simulink model "controller"  (R2021b)
settings: Solver=ode4  StartTime=0.0  StopTime=10.0  FixedStep=0.001  RelTol=1e-3
undefined symbols (not defined in the file): B, J, K2, K3, Kb, Kt, L, L1, L2, L3, R, Ts
settings Model: Creator=user  LastModifiedBy=user

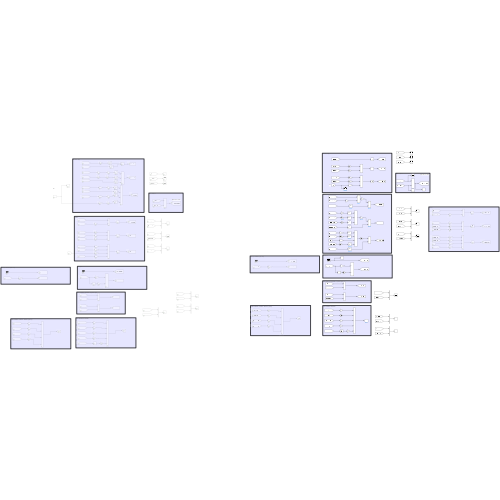
[thumbnail: Simulink's stored preview of the top-level diagram]
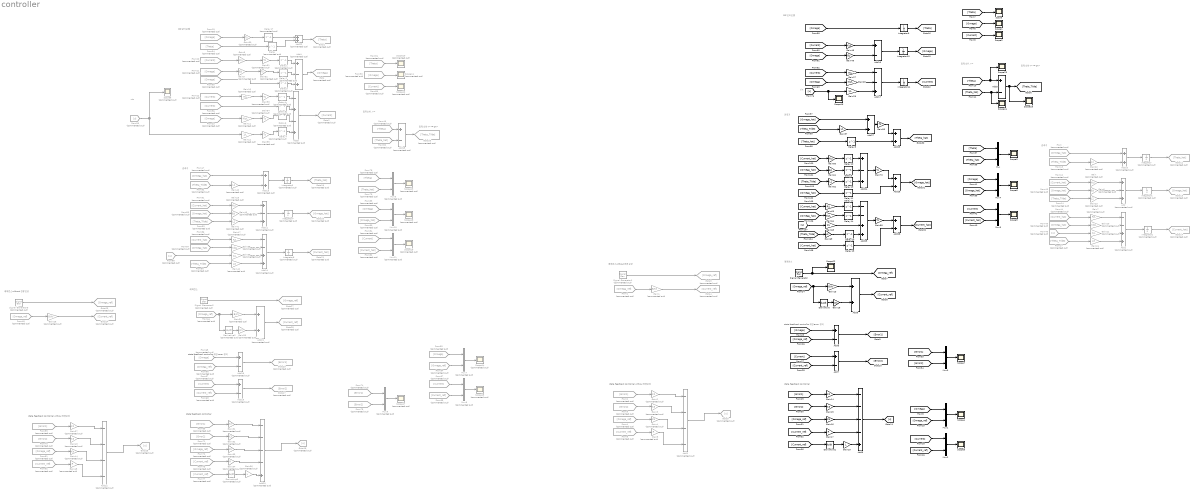
== system controller ==
  note: 관측기
  note: vin
  note: DC 모터 모델
  note: state feedback controller
  note: 레퍼런스
  note: state feedback controller 위한 error 정의
  note: 레퍼런스 without 전류 보상
  note: state feedback controller without 전류보상
  note: 출력 오차 Y~ = CX~
  note: 출력 오차, Y~
  note: 관측기
  note: vin
  note: state feedback controller
  note: 관측기
  note: 출력 오차 Y~ = CX~
  note: 레퍼런스 without 전류 보상
  note: 출력 오차, Y~
  note: DC 모터 모델
  note: state feedback controller without 전류보상
  note: state feedback controller 위한 error 정의
  note: 레퍼런스
  Add : Sum  Commented=on  Inputs=+-+
  Add1 : Sum  Commented=on  Inputs=----
  Add{10,13,21..22} (4 alike) : Sum  Commented=on
  Add11 : Sum  Commented=on  Inputs=+-+
  Add12 : Sum  Commented=on  Inputs=----
  Add14 : Sum  Commented=on  Inputs=--++
  Add15 : Sum  Commented=on  Inputs=+-
  Add{3,6..7,16} (4 alike) : Sum  Inputs=+-
  Add17 : Sum  Inputs=--+
  Add18 : Sum  Commented=on  Inputs=+-
  Add19 : Sum  Commented=on  Inputs=+-
  Add2 : Sum  Commented=on  Inputs=--++
  Add20 : Sum  Commented=on  Inputs=----+
  Add{9,23,26..28} (5 alike) : Sum
  Add24 : Sum  Inputs=+-+
  Add25 : Sum  Inputs=--++
  Add4 : Sum  Commented=on  Inputs=+-+
  Add5 : Sum  Commented=on  Inputs=-+-+
  Add8 : Sum  Inputs=----+
  Delay : Delay  Commented=on  DelayLength=1  InitialCondition=0
  Delay{1..7,17} (8 alike) : Delay  Commented=on  DelayLength=1
  Delay{8..14,19..20} (9 alike) : Delay  DelayLength=1
  Derivative : Derivative
  Derivative1 : Derivative
  Derivative2 : Derivative  Commented=on
  Derivative3 : Derivative  Commented=on
  From{,43,45,47,80,85,87} (7 alike) : From  Commented=on  GotoTag=Omega_hat
  From{1,4,48,54,64,66,72,81} (8 alike) : From  Commented=on  GotoTag=Omega_ref
  From{12,44,51,82,86} (5 alike) : From  Commented=on  GotoTag=Current_hat
  From{13..14,17,52..53,56} (6 alike) : From  Commented=on  GotoTag=Theta_Tilde
  From{19,21,23,65,83,90,93,95} (8 alike) : From  Commented=on  GotoTag=Omega
  From{2,59,69,74} (4 alike) : From  Commented=on  GotoTag=Error1
  From{20,22,57,67,84,89,96} (7 alike) : From  Commented=on  GotoTag=Current
  From{3,70..71,75} (4 alike) : From  Commented=on  GotoTag=Error2
  From35 : From  Commented=on  GotoTag=u
  From46 : From  Commented=on  GotoTag=u
  From{49,78,91,94} (4 alike) : From  Commented=on  GotoTag=Theta
  From50 : From  Commented=on  GotoTag=Theta_hat
  From{8,55,68,73,77,92} (6 alike) : From  Commented=on  GotoTag=Current_ref
  From79 : From  Commented=on  GotoTag=Theta_hat
  From88 : From  Commented=on  GotoTag=u
  Gain : Gain  Commented=on  Gain=Kt/J
  Gain1 : Gain  Commented=on  Gain=B/Kt
  Gain10 : Gain  Commented=on  Gain=R/L
  Gain11 : Gain  Commented=on  Gain=Kb/L
  Gain12 : Gain  Commented=on  Gain=1/L
  Gain13 : Gain  Gain=B/Kt
  Gain14 : Gain  Gain=K2
  Gain15 : Gain  Gain=K3
  Gain16 : Gain  Gain=Kb
  Gain17 : Gain  Gain=R
  Gain18 : Gain  Gain=J/Kt
  Gain19 : Gain  Gain=L
  Gain2 : Gain  Commented=on  Gain=K2
  Gain20 : Gain  Commented=on  Gain=Kb/L
  Gain21 : Gain  Commented=on  Gain=1/L
  Gain22 : Gain  Commented=on  Gain=L1
  Gain23 : Gain  Commented=on  Gain=L2
  Gain24 : Gain  Commented=on  Gain=L3
  Gain25 : Gain  Commented=on  Gain=Kt/J
  Gain26 : Gain  Commented=on  Gain=B/Kt
  Gain27 : Gain  Gain=R/L
  Gain28 : Gain  Gain=Kb/L
  Gain29 : Gain  Gain=1/L
  Gain3 : Gain  Commented=on  Gain=K3
  Gain30 : Gain  Commented=on  Gain=B/Kt
  Gain31 : Gain  Commented=on  Gain=K2
  Gain32 : Gain  Commented=on  Gain=K3
  Gain33 : Gain  Commented=on  Gain=Kb
  Gain34 : Gain  Commented=on  Gain=R
  Gain35 : Gain  Commented=on  Gain=J/Kt
  Gain36 : Gain  Commented=on  Gain=L
  Gain37 : Gain  Commented=on  Gain=K2
  Gain38 : Gain  Commented=on  Gain=Kb/L
  Gain39 : Gain  Commented=on  Gain=1/L
  Gain4 : Gain  Commented=on  Gain=Kb
  Gain40 : Gain  Commented=on  Gain=L1
  Gain41 : Gain  Commented=on  Gain=L2
  Gain42 : Gain  Commented=on  Gain=L3
  Gain43 : Gain  Commented=on  Gain=K3
  Gain44 : Gain  Commented=on  Gain=Kb
  Gain45 : Gain  Commented=on  Gain=R
  Gain46 : Gain  Commented=on  Gain=B/J
  Gain47 : Gain  Commented=on  Gain=R/L
  Gain48 : Gain  Gain=Kt/J
  Gain49 : Gain  Gain=B/J
  Gain5 : Gain  Commented=on  Gain=R
  Gain{50..55} (6 alike) : Gain  Commented=on  Gain=Ts
  Gain56 : Gain  Gain=Ts
  Gain57 : Gain  Gain=L1
  Gain58 : Gain  Gain=Ts
  Gain6 : Gain  Commented=on  Gain=B/J
  Gain60 : Gain  Gain=Kt/J
  Gain61 : Gain  Gain=B/J
  Gain62 : Gain  Gain=L2
  Gain63 : Gain  Gain=R/L
  Gain64 : Gain  Gain=Kb/L
  Gain65 : Gain  Gain=1/L
  Gain69 : Gain  Gain=L3
  Gain7 : Gain  Commented=on  Gain=R/L
  Gain70 : Gain  Gain=Ts
  Gain8 : Gain  Commented=on  Gain=Kt/J
  Gain9 : Gain  Commented=on  Gain=B/J
  Goto : Goto  Commented=on  GotoTag=Omega
  Goto1 : Goto  Commented=on  GotoTag=Theta
  Goto12 : Goto  Commented=on  GotoTag=Theta_hat
  Goto13 : Goto  Commented=on  GotoTag=Omega_hat
  Goto14 : Goto  Commented=on  GotoTag=Current_hat
  Goto17 : Goto  Commented=on  GotoTag=Error2
  Goto18 : Goto  Commented=on  GotoTag=u
  Goto19 : Goto  Commented=on  GotoTag=Theta_hat
  Goto2 : Goto  Commented=on  GotoTag=Current
  Goto20 : Goto  Commented=on  GotoTag=Omega_hat
  Goto21 : Goto  Commented=on  GotoTag=Current_hat
  Goto23 : Goto  Commented=on  GotoTag=Omega_ref
  Goto24 : Goto  Commented=on  GotoTag=Current_ref
  Goto25 : Goto  Commented=on  GotoTag=u
  Goto26 : Goto  Commented=on  GotoTag=Theta_Tilde
  Goto27 : Goto  Commented=on  GotoTag=Omega_ref
  Goto28 : Goto  Commented=on  GotoTag=Current_ref
  Goto29 : Goto  Commented=on  GotoTag=Error1
  Goto3 : Goto  Commented=on  GotoTag=Omega_ref
  Goto4 : Goto  Commented=on  GotoTag=Current_ref
  Goto5 : Goto  Commented=on  GotoTag=u
  Integrator{,1..2,6..8} (6 alike) : Integrator  Commented=on
  Integrator10 : Integrator
  Integrator11 : Integrator
  Integrator9 : Integrator  InitialCondition=1
  Mux{,1..5} (6 alike) : Mux  Inputs=2
  Mux{6..11} (6 alike) : Mux  Commented=on  Inputs=2
  Scope{,1..5,7..9,16,22..25} (14 alike) : Scope
  Scope{6,10..15,17..19} (10 alike) : Scope  Commented=on
  Signal Generator : SignalGenerator  Units=rad/sec
  Signal Generator1 : SignalGenerator  Commented=on  Units=rad/sec
  Signal Generator2 : SignalGenerator  Commented=on  Units=rad/sec
  Signal Generator3 : SignalGenerator  Commented=on  Units=rad/sec
  wires:
  Add22/1 -> Goto1/1
  From19/1 -> Gain50/1
  From23/1 -> Gain11/1
  From20/1 -> Gain8/1
  From21/1 -> Gain9/1
  From22/1 -> Gain10/1
  Gain8/1 -> Gain51/1
  Gain9/1 -> Gain52/1
  [Current] -> Scope2/1
  [Omega] -> Scope1/1
  [Theta] -> Scope/1
  From35/1 -> Scope6/1, Gain12/1
  [Current_ref] -> Derivative1/1
  Gain19/1 -> Add8/5
  Derivative1/1 -> Gain19/1
  Gain17/1 -> Add8/4
  [Omega_ref] -> Add6/2
  [Current] -> Add7/1
  Gain18/1 -> Add9/2
  Mux3/1 -> Scope7/1
  Gain13/1 -> Add9/1
  [Omega_ref] -> Gain13/1, Derivative/1
  [Error1] -> Gain14/1
  Add9/1 -> [Current_ref]
  Derivative/1 -> Gain18/1
  Signal Generator/1 -> Scope22/1, [Omega_ref]
  [Error1] -> Mux3/1
  Gain16/1 -> Add8/3
  [Error2] -> Mux3/2
  [Error2] -> Gain15/1
  Add8/1 -> [u]
  Gain14/1 -> Add8/1
  [Current_ref] -> Gain17/1
  Add6/1 -> [Error1]
  Gain15/1 -> Add8/2
  [Omega_ref] -> Gain16/1
  [Current_ref] -> Add7/2
  Add7/1 -> [Error2]
  [Omega] -> Add6/1
  [Current] -> Mux2/1
  Mux2/1 -> Scope5/1
  [Current_ref] -> Mux2/2
  [Omega_ref] -> Mux1/2
  Mux1/1 -> Scope4/1
  Signal Generator1/1 -> Goto3/1
  From1/1 -> Gain1/1
  Gain1/1 -> Goto4/1
  Gain3/1 -> Add1/2
  From8/1 -> Gain5/1
  From4/1 -> Gain4/1
  From3/1 -> Gain3/1
  Add1/1 -> Goto5/1
  Gain2/1 -> Add1/1
  Gain4/1 -> Add1/3
  From2/1 -> Gain2/1
  Gain5/1 -> Add1/4
  [Omega] -> Mux1/1
  [Theta] -> Scope23/1, Add3/1
  [Theta_hat] -> Scope24/1, Add3/2
  [Theta_hat] -> Mux/2
  [Theta] -> Mux/1
  Gain6/1 -> Add/2
  Mux4/1 -> Scope8/1
  [Current_hat] -> Mux5/2
  Gain24/1 -> Add2/4
  Gain22/1 -> Add10/2
  Mux5/1 -> Scope9/1
  Gain23/1 -> Add/3
  [Omega] -> Mux4/1
  From/1 -> Add10/1
  From14/1 -> Gain23/1
  Integrator2/1 -> Goto14/1
  Add10/1 -> Integrator/1
  Integrator1/1 -> Goto13/1
  Gain7/1 -> Add2/1
  From12/1 -> Gain/1
  Gain21/1 -> Add2/3
  Add/1 -> Integrator1/1
  Mux/1 -> Scope3/1
  Add2/1 -> Integrator2/1
  From44/1 -> Gain7/1
  From17/1 -> Gain24/1
  From13/1 -> Gain22/1
  From45/1 -> Gain20/1
  [Omega_hat] -> Mux4/2
  Gain/1 -> Add/1
  From43/1 -> Gain6/1
  [Current] -> Mux5/1
  Gain20/1 -> Add2/2
  Integrator/1 -> Goto12/1
  From46/1 -> Gain21/1
  Gain47/1 -> Add14/1
  From56/1 -> Gain42/1
  Gain49/1 -> Add16/2
  Add13/1 -> Integrator6/1
  From50/1 -> Add15/2
  Integrator7/1 -> Goto20/1
  Add16/1 -> Integrator10/1
  Gain36/1 -> Add20/5
  From55/1 -> Mux8/2
  Gain41/1 -> Add11/3
  Mux11/1 -> Scope19/1
  From81/1 -> Gain44/1
  Gain26/1 -> Goto24/1
  From82/1 -> Mux11/2
  Add20/1 -> Goto18/1
  From77/1 -> Derivative3/1
  Gain40/1 -> Add13/2
  From93/1 -> Mux7/1
  Gain42/1 -> Add14/4
  Gain46/1 -> Add11/2
  From70/1 -> Gain43/1
  Gain37/1 -> Add12/1
  Gain31/1 -> Add20/1
  From71/1 -> Gain32/1
  Add12/1 -> Goto25/1
  From48/1 -> Gain26/1
  From65/1 -> Add18/1
  From57/1 -> Mux8/1
  Gain27/1 -> Add17/1
  From75/1 -> Mux9/2
  From92/1 -> Gain45/1
  Gain43/1 -> Add12/2
  From54/1 -> Mux7/2
  Gain32/1 -> Add20/2
  Mux8/1 -> Scope15/1
  Add19/1 -> Goto17/1
  Add17/1 -> Integrator11/1
  Gain30/1 -> Add21/1
  Derivative3/1 -> Gain36/1
  Gain48/1 -> Add16/1
  Add18/1 -> Goto29/1
  Add21/1 -> Goto28/1
  Integrator11/1 -> [Current]
  [Omega] -> Gain28/1
  Gain28/1 -> Add17/2
  [Current] -> Gain48/1
  Gain29/1 -> Add17/3
  From91/1 -> Scope10/1
  Gain44/1 -> Add12/3
  From68/1 -> Add19/2
  Signal Generator2/1 -> Goto27/1
  Integrator9/1 -> [Theta]
  From72/1 -> Gain33/1
  Derivative2/1 -> Gain35/1
  From49/1 -> Add15/1
  Integrator6/1 -> Goto19/1
  Integrator10/1 -> [Omega]
  Signal Generator3/1 -> Goto23/1
  From89/1 -> Scope12/1
  Mux6/1 -> Scope13/1
  From78/1 -> Mux6/1
  From53/1 -> Gain41/1
  Gain35/1 -> Add21/2
  Gain45/1 -> Add12/4
  From59/1 -> Gain37/1
  From67/1 -> Add19/1
  From66/1 -> Add18/2
  Add11/1 -> Integrator7/1
  [u] -> Scope16/1, Gain29/1
  From84/1 -> Mux11/1
  [Omega] -> Integrator9/1
  From88/1 -> Gain39/1
  Mux10/1 -> Scope18/1
  [Omega] -> Gain49/1
  From52/1 -> Gain40/1
  From64/1 -> Gain30/1, Derivative2/1
  Integrator8/1 -> Goto21/1
  Gain39/1 -> Add14/3
  From51/1 -> Gain25/1
  From69/1 -> Gain31/1
  From87/1 -> Gain38/1
  From73/1 -> Gain34/1
  From90/1 -> Scope11/1
  [Current] -> Gain27/1
  Gain25/1 -> Add11/1
  Gain38/1 -> Add14/2
  From85/1 -> Gain46/1
  Mux7/1 -> Scope14/1
  From47/1 -> Add13/1
  From80/1 -> Mux10/2
  Gain33/1 -> Add20/3
  From79/1 -> Mux6/2
  From83/1 -> Mux10/1
  Gain34/1 -> Add20/4
  Add15/1 -> Goto26/1
  From86/1 -> Gain47/1
  Mux9/1 -> Scope17/1
  Add14/1 -> Integrator8/1
  From74/1 -> Mux9/1
  From94/1 -> Delay/1
  Delay/1 -> Add22/2
  From95/1 -> Delay3/1
  Gain52/1 -> Delay2/1
  Gain51/1 -> Delay1/1
  Delay1/1 -> Add4/1
  Delay2/1 -> Add4/2
  Delay3/1 -> Add4/3
  Add4/1 -> Goto/1
  Gain10/1 -> Gain53/1
  Gain53/1 -> Delay4/1
  From96/1 -> Delay5/1
  Gain11/1 -> Gain54/1
  Gain54/1 -> Delay6/1
  Gain12/1 -> Gain55/1
  Gain55/1 -> Delay7/1
  Delay4/1 -> Add5/1
  Delay5/1 -> Add5/2
  Delay6/1 -> Add5/3
  Delay7/1 -> Add5/4
  Add5/1 -> Goto2/1
  [Theta_hat] -> Delay8/1
  Delay8/1 -> Add23/2
  [Theta_Tilde] -> Gain57/1
  Add23/1 -> [Theta_hat]
  Add24/1 -> Gain70/1
  [Omega_hat] -> Gain61/1
  [Omega_hat] -> Delay11/1
  [Current_hat] -> Gain60/1
  [Theta_Tilde] -> Gain62/1
  [Current_hat] -> Gain63/1
  [Omega_hat] -> Gain64/1
  [Theta_Tilde] -> Gain69/1
  Gain69/1 -> Delay20/1
  [u] -> Gain65/1
  Gain50/1 -> Delay17/1
  Delay17/1 -> Add22/1
  Delay20/1 -> Add25/4
  Gain56/1 -> Add23/1
  Gain63/1 -> Delay12/1
  Gain64/1 -> Delay14/1
  Delay9/1 -> Add24/2
  Delay10/1 -> Add24/1
  Delay12/1 -> Add25/1
  [Omega_hat] -> Add27/1
  Add27/1 -> Gain56/1
  Gain57/1 -> Add27/2
  Add3/1 -> Scope25/1, [Theta_Tilde]
  Gain62/1 -> Delay19/1
  Delay19/1 -> Add24/3
  Gain70/1 -> Add26/1
  Delay11/1 -> Add26/2
  Add26/1 -> [Omega_hat]
  Gain60/1 -> Delay10/1
  Gain61/1 -> Delay9/1
  [Current_hat] -> Delay13/1
  Delay14/1 -> Add25/2
  Gain58/1 -> Add28/1
  Gain65/1 -> Add25/3
  Add25/1 -> Gain58/1
  Delay13/1 -> Add28/2
  Add28/1 -> [Current_hat]
